simulink model "PIC32MZ_EF_CuriosityBoard_SHT1x_ExtMode"  (R2016b)
settings: Solver=FixedStepDiscrete  StartTime=0.0  StopTime=inf  FixedStep=0.01  RelTol=1e-3
undefined symbols (not defined in the file or in its folder): A14, A15, B0, B1, B5, C2, C3, D1, D2, D3, DiscIntNeverNeededParam, F5, Max, ms, NumBits1, NumBits2, OC3max, OC4max, OC5max, Pin, Resol, Timer, us
libraries: MCHP_Blockset x14, simulink x6
settings Model: SimulationMode=external  ExtModeBatchMode=on  ExtModeTrigDuration=1  Creator=M91449  LastModifiedBy=Lubin Kerhuel
settings OptimizationCC: DefaultParameterBehavior=Inlined  UseSpecifiedMinMax=on  ZeroExternalMemoryAtStartup=off  ZeroInternalMemoryAtStartup=off  NoFixptDivByZeroProtection=on  EfficientFloat2IntCast=on
settings DebuggingCC: ParameterTunabilityLossMsg=error
settings HardwareCC: ProdBitPerPointer=32  ProdBitPerSizeT=32  ProdBitPerPtrDiffT=32  ProdLargestAtomicInteger=Integer  ProdWordSize=32  ProdLongLongMode=on  ProdHWDeviceType=Generic->Custom
settings ModelReferenceCC: ModelReferenceNumInstancesAllowed=Single
settings RTWCC: SystemTargetFile=MCHP_pic32_stf.tlc  TemplateMakefile=MCHP_pic32.tmf  Description=Microchip Embedded Target PIC32 (real-time)  GenerateReport=on  IncludeHyperlinkInReport=on  LaunchReport=on  GenerateTraceInfo=on  GenerateTraceReport=on  GenerateTraceReportSl=on  GenerateTraceReportSf=on  GenerateTraceReportEml=on
settings CodeAppCC: ForceParamTrailComments=on  IgnoreCustomStorageClasses=off  MaxIdLength=255  OperatorAnnotations=on  SimulinkDataObjDesc=on  SFDataObjDesc=on  MATLABFcnDesc=on  InsertBlockDesc=on  MATLABSourceComments=on
settings STFCustomTargetCC: TargetLibSuffix=_lib.a  TargetLangStandard=C99 (ISO)  IncludeMdlTerminateFcn=off  CombineOutputUpdateFcns=on  CombineSignalStateStructs=on  ERTCustomFileBanners=on  SupportContinuousTime=off  RemoveResetFunc=on  MATLABClassNameForMDSCustomization=Simulink.SoftwareTarget.ERTCustomization  GRTInterface=off  SystemTargetFile=MCHP_pic32_stf.tlc
settings ERTTargetCC: TargetLibSuffix=_lib.a  TargetLangStandard=C99 (ISO)  ParMdlRefBuildCompliant=off  CompOptLevelCompliant=off  ConcurrentExecutionCompliant=off  IncludeMdlTerminateFcn=off  CombineSignalStateStructs=on  ERTFirstTimeCompliant=off  SupportNonInlinedSFcns=on  ModelStepFunctionPrototypeControlCompliant=off  CPPClassGenCompliant=off  UseToolchainInfoCompliant=off  ExtMode=on  ExtModeStaticAllocSize=512  ExtModeMexFile=ext_serial_win32_comm_no_acks  ExtModeMexArgs=1 9 115200  InlinedParameterPlacement=NonHierarchical  ERTSrcFileBannerTemplate=MCHP_dsPIC_code_template.cgt  ERTHdrFileBannerTemplate=MCHP_dsPIC_code_template.cgt  ERTDataSrcFileTemplate=MCHP_dsPIC_code_template.cgt  ERTDataHdrFileTemplate=MCHP_dsPIC_code_template.cgt  ERTCustomFileTemplate=MCHP_main.tlc

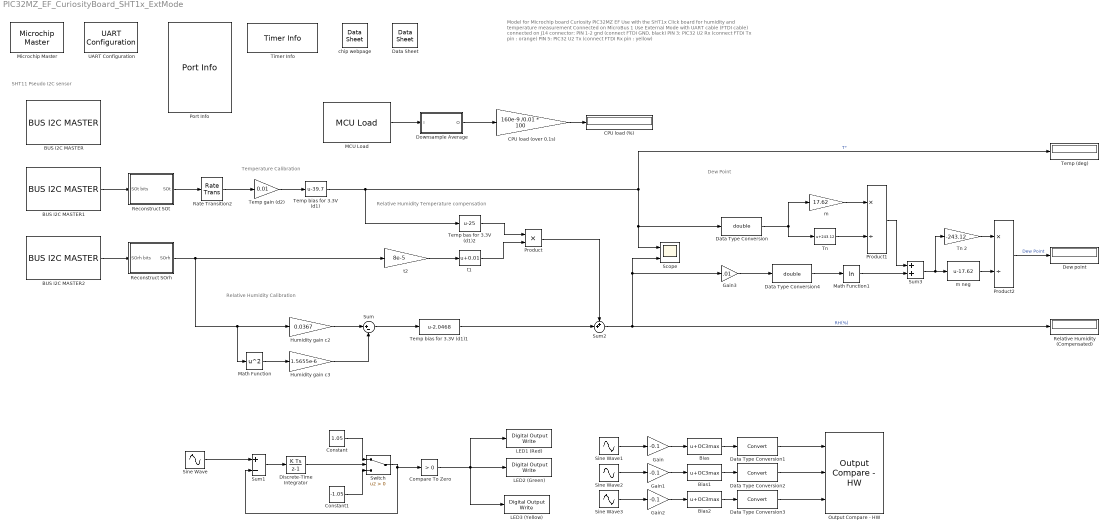
== system PIC32MZ_EF_CuriosityBoard_SHT1x_ExtMode ==
  note: Model for Microchip board Curiosity PIC32MZ EF
      | Use with the SHT1x Click board for humidity and temperature measurement
      | Connected on MicroBus 1
      |
      | Use External Mode with UART cable (FTDI cable) connected on J14 connector:
      | PIN 1-2 gnd (connect FTDI GND, black)
      | PIN 3: PIC32 U2 Rx (connect FTDI Tx pin : orange)
      | PIN 5: PIC32 U2 Tx (connect FTDI Rx pin : yellow)
  note: SHT11 Pseudo I2C sensor
  note: Dew Point
  note: Relative Humidity Temperature compensation
  note: Relative Humidity Calibration
  note: Temperature Calibration
  BUS I2C MASTER : MCHP_Blockset/BUS I2C/BUS I2C MASTER  I2CRef=1  I2C_IntPriority=5  I2Csequence_txt="Initial-Configuration$     ---     $Start    % SHT11 humidity sensor does not use standard I2C protocol$Stop$Start$Write Data (x1)  Write:{[0x03]}      % Start temperature meas (14 bit, might take up to 320ms)$     ---         % Must wait 320ms (sensor pull down SDA line when done)"  I2Csequence_num=[BFF0000000000000 40E0000000000000 40F86A0000000000 40F8650105EF3846]$4070000000000000$[3FF0000000000000 40E0000000000000 40F86A0000000000 40F8650105EF3846]$[4000000000000000 40E0000000000000 40F86A0000000000 40F8650105EF3846]$[3FF0000000000000 40E0000000000000 40F86A0000000000 40F8650105EF3846]$[4050000000000000 3FF0000000000000 0000000000000000 4008000000000000]$4070000000000000  InitialConfigurationNum=0  PIN_SDA_TXT=A15 / Pin[67]  PIN_SCL_TXT=A14 / Pin[66]  S_INPUT="[5  5]"  S_OUTPUT=[5]  S_INPUT_Size="[2  2]"  S_OUTPUT_Size=[4]  BlockingMode=off  SequenceCompleted=off  SampleTime=[1 ]  MCHP_MASTERLINK=PIC32MZ_EF_CuriosityBoard_SHT1x_ExtMode/Microchip Master  MCHP_PORT={I2C 1 Clock}{SCL1}13:0:A14;{I2C 1 SDA}{SDA1}13:0:A15;  ORDERING=0
  BUS I2C MASTER1 : MCHP_Blockset/BUS I2C/BUS I2C MASTER  I2CRef=1  I2C_IntPriority=5  I2Csequence_txt="Initial-Configuration$     ---     $Read Data (x3)  Read:{Out 3}    % Read 14 bit temperature (0.01 deg), last byte is CRC$Stop$Start    % Start measurement for humidity$Stop$Start$Write Data (x1)  Write:{[0x05]}      % Must wait up to 80 ms (12 bit resolution)"  I2Csequence_num=[BFF0000000000000 40E0000000000000 40F86A0000000000 40F8650105EF3846]$4070000000000000$[4060000000000000 4008000000000000]$[4000000000000000 40E0000000000000 40F86A0000000000 40F8650105EF3846]$[3FF0000000000000 40E0000000000000 40F86A0000000000 40F8650105EF3846]$[4000000000000000 40E0000000000000 40F86A0000000000 40F8650105EF3846]$[3FF0000000000000 40E0000000000000 40F86A0000000000 40F8650105EF3846]$[4050000000000000 3FF0000000000000 0000000000000000 4014000000000000]  InitialConfigurationNum=0  PIN_SDA_TXT=A15 / Pin[67]  PIN_SCL_TXT=A14 / Pin[66]  S_INPUT="[5  5]"  S_OUTPUT=[5]  S_INPUT_Size="[2  2]"  S_OUTPUT_Size=[4]  BlockingMode=off  SequenceCompleted=off  SampleTime=[1 0.640]  MCHP_MASTERLINK=PIC32MZ_EF_CuriosityBoard_SHT1x_ExtMode/Microchip Master  MCHP_PORT={I2C 1 Clock}{SCL1}13:0:A14;{I2C 1 SDA}{SDA1}13:0:A15;  ORDERING=0
  BUS I2C MASTER2 : MCHP_Blockset/BUS I2C/BUS I2C MASTER  I2CRef=1  I2C_IntPriority=5  I2Csequence_txt="Initial-Configuration$     ---     $Read Data (x3)  Read:{Out 3}    % Read humidity$Stop"  I2Csequence_num=[BFF0000000000000 40E0000000000000 40F86A0000000000 40F8650105EF3846]$[4070000000000000]$[4060000000000000 4008000000000000]$[4000000000000000 40E0000000000000 40F86A0000000000 40F8650105EF3846]  InitialConfigurationNum=0  PIN_SDA_TXT=A15 / Pin[67]  PIN_SCL_TXT=A14 / Pin[66]  S_INPUT="[5  5]"  S_OUTPUT=[5]  S_INPUT_Size="[2  2]"  S_OUTPUT_Size=[4]  BlockingMode=off  SequenceCompleted=off  SampleTime=[1 .800]  MCHP_MASTERLINK=PIC32MZ_EF_CuriosityBoard_SHT1x_ExtMode/Microchip Master  MCHP_PORT={I2C 1 Clock}{SCL1}13:0:A14;{I2C 1 SDA}{SDA1}13:0:A15;  ORDERING=0
  Bias : Bias  Bias=OC3max
  Bias1 : Bias  Bias=OC3max
  Bias2 : Bias  Bias=OC3max
  CPU load (over 0.1s) : Gain  Gain=160e-9 /0.01 * 100  OutDataTypeStr=double
  CPU load (%) : Display
  Compare To Zero : simulink/Logic and Bit Operations/Compare To Zero  relop=>  OutDataTypeStr=boolean
  Constant : Constant  Value=1.05
  Constant1 : Constant  Value=-1.05
  Data Sheet : MCHP_Blockset/System Info/Data Sheet  DOC_Type=datasheet  DOC_MCHP_Id=32MZ2048EFM100_datasheet  DOC_FilePath=C:\Users\M91449\AppData\Local\Temp\PIC32MZ-EF- Family-DS60001320F.pdf  DOC_FileLastCheckTime="[2019              8             26             15             22         57.115]"  cpy_MCHP_Id=32MZ2048EFM100  MCHP_MASTERLINK=PIC32MZ_EF_CuriosityBoard_SHT1x_ExtMode/Microchip Master
      settings: AttributesFormatString=%<cpy_MCHP_Id>
  Data Type Conversion : DataTypeConversion  OutDataTypeStr=double
  Data Type Conversion1 : DataTypeConversion
  Data Type Conversion2 : DataTypeConversion
  Data Type Conversion3 : DataTypeConversion
  Data Type Conversion4 : DataTypeConversion  OutDataTypeStr=double
  Dew point : Display
  Discrete-Time Integrator : DiscreteIntegrator  gainval=1  InitialConditionSetting=State (most efficient)  SampleTime=-1  ICPrevOutput=DiscIntNeverNeededParam  ICPrevScaledInput=DiscIntNeverNeededParam
  Downsample Average : Subsystem  mask{InputSampleTime=.01, DownSample=100}
      mask prompts: InputSampleTime "Input sample time"; DownSample "DownSample Factor"
      mask Display: disp([ 'DwnSmp\n1/' get_param(gcb,'DownSample')]);
  Gain : Gain  Gain=-0.1
  Gain1 : Gain  Gain=-0.1
  Gain2 : Gain  Gain=-0.1
  Gain3 : Gain  Gain=.01  OutMin=[0]  OutMax=[1]  OutDataTypeStr=fixdt(1,32)
  Humidity gain c2 : Gain  Gain=0.0367  OutMax=2^16*0.0367  OutDataTypeStr=fixdt(1,32)
  Humidity gain c3 : Gain  Gain=1.5655e-6  OutMax=2^32*1.5655e-6  OutDataTypeStr=fixdt(0,32)
  LED1 (Red) : MCHP_Blockset/Digital IO/Digital Output Write  PORT=Dynamic Options  PORT_TXT="E   [ 0 : 9 ]"  PIN=3  PACK=off  SIMULTANEOUS=off  ORDERING=None  SampleTime=-1  MCHP_PORT={Digital Out}{DOU}1:1:E3;  MCHP_MASTERLINK=PIC32MZ_EF_CuriosityBoard_SHT1x_ExtMode/Microchip Master
  LED2 (Green) : MCHP_Blockset/Digital IO/Digital Output Write  PORT=Dynamic Options  PORT_TXT="E   [ 0 : 9 ]"  PIN=4  PACK=off  SIMULTANEOUS=off  ORDERING=None  SampleTime=-1  MCHP_PORT={Digital Out}{DOU}1:1:E4;  MCHP_MASTERLINK=PIC32MZ_EF_CuriosityBoard_SHT1x_ExtMode/Microchip Master
  LED3 (Yellow) : MCHP_Blockset/Digital IO/Digital Output Write  PORT=Dynamic Options  PORT_TXT="E   [ 0 : 9 ]"  PIN=6  PACK=off  SIMULTANEOUS=off  ORDERING=None  SampleTime=-1  MCHP_PORT={Digital Out}{DOU}1:1:E6;  MCHP_MASTERLINK=PIC32MZ_EF_CuriosityBoard_SHT1x_ExtMode/Microchip Master
  MCU Load : MCHP_Blockset/Profiling/MCU Load  MCULoadPin=Dynamic Options  MCULoadPin_TXT=F5 / Pin[65]  MCULoadMeasure=on  TIMER_Resolution=Dynamic Options  TIMER_Resolution_TXT="Resol: 0.16(us)  -  Max: 10.5(ms)"  MCHP_PORT={MCU Load Pin}{MCU_Load}0:1:F5;  MCHP_TIMER_REQUEST={MCU_Load}{MCU_Load}21:5:0:0:[]:1048576;  MCHP_TIMER_RESULT=[4 65535 ]  MCHP_MASTERLINK=PIC32MZ_EF_CuriosityBoard_SHT1x_ExtMode/Microchip Master  MCHP_COMPILED_INFO="CompiledSampleTime= [0.01   0 ];CompiledInportDataTypes=[ ];CompiledInportDataWidth=[];"  Info="Timer 4:  Resol: 160(ns)  -  Max: 10.4858(ms)"  SampleTime=.01
  Math Function : Math  Operator=square  OutDataTypeStr=Inherit: Inherit via internal rule
  Math Function1 : Math  Operator=log  OutDataTypeStr=Inherit: Inherit via internal rule
  Microchip Master : MCHP_Blockset/System Configuration/Microchip Master  Priority=1  PICREF=32MZ2048EFM100  TIMESTEP_REF="Timer  ( 0.01s )"  BUSYFLAG=Dynamic Options  BUSYFLAG_TXT=None  PWRTEN=Not used  BOREN=Disable  BODENV=2.7V  BORV=Not used  FPWRT=128ms  DSBOREN=Enable ZPBOR during Deep Sleep Mode  DSLPBOR=Not used  MCLRE=Enabled  SMCLR=MCLR pin generates a normal system Reset  PMDL1WAY=Allow only one reconfiguration  RSTPRI=Device will obtain reset instruction from Primary flash  TEMP=Not used  SOSCSRC=Not used  SOSCSEL=Not used  IOL1WAY=Allow only one reconfiguration  ALTVREF=Not used  DISUVREG=Not used  DSSWEN=Not used  LPCFG=Not used  RTCBAT=Not used  VBTBOR=Not used  WUTSEL=Not used  POWERSAVE=off  FNOSC=Primary Osc (HS;EC)  FPR=ECIO w/ PLL 16x  FOSFPR=HS3 w/PLL 16x  FOS=Primary Oscillator  FRANGE=High Range  OSCILLATOR_SELECT=External Clock  OSCILLATOR_SELECT_spd=External Clock  QUARTZ=24e6  QUARTZ_spd=24e6  POSCGAIN=2x gain setting  POSCBOOST=Boost the kick start of the oscillator  SOSCGAIN=2x gain setting  SOSCBOOST=Boost the kick start of the oscillator  ACTIV_PLL=on  ACTIV_PLL_spd=on  MIPS_DESIRED=200e6  MIPS_DESIRED_spd=200e6  FPLLMUL=Not used  FPLLIDIV=3x Divider  POSCFREQ=Not used  POSCMD=Primary Oscillator Disabled  POSCMOD=External clock mode  MIPS=199.99999999999997 * 1e6  ACLKCON=Optimized for PWM resolution & ADC conversion speed  ACLKCON_spd=Optimized for PWM resolution & ADC conversion speed  FPLLODIV=2x Divider  PLLKEN=Clock switch to PLL source will wait until the PLL lock signal is valid.  FCKSM=Clock Switch Enabled; FSCM Enabled  FCKSMEN=Sw Disabled; Mon Disabled  IESO=Enabled  DSWDTPS=1:2^36  FWDTEN=Disable  FWDTWINSZ=Window size is 25%  FWPSA=1:512  FWPSA0=1:128  FWPSB=1:16  WDT=Disable  WDTPOST=1:32768  WDTPRE=1:128  WDTPS=1:1048576  WINDIS=Watchdog Timer is in non-Window mode  WWDTEN=Non-Window mode  DSWDTEN=Enable DSWDT during Deep Sleep Mode  DSWDTOSC=Select LPRC as DSWDT Reference clock  FPBDIV=Not used  FSOSCEN=Disable Secondary Oscillator  LPRCSEL=Not used  OSCIOFCN=Not used  OSCIOFNC=Disable  LVRCFG=Not used  PLL_96MHZ=Not used  PLL96MHZ=Not used  PLLDIV=Not used  WDTCLK=Not used  WDTCMX=Not used  WDTWIN=Watchdog Window is 25% of WDT period  XTCFG=24-32 MHz crystals  XTBST=Boost the kick-start  APL=Aux Flash Code protect is disabled  APLK=Aux Flash Write Protection or Code Protection is Enabled  AWRP=Aux Flash may be written  BSS=No Boot program Flash segment  BWP=Not used  BWRP=Boot Segment may be written  CP=Protection Disabled  EBS=No Boot EEPROM  ESS=No Segment Data EEPROM  GCP=General Segment Code protect is Disabled  GSS=User program memory is not code-protected  GSS0=Not used  GSSK=General Segment Write Protection or Code Protection is Enabled  GWRP=General Segment may be written  PWP=Not used  RBS=No Boot RAM  RSS=No Secure RAM  SSS=No Secure Segment  SWRP=Secure segment may be written  WPCFG=Not used  WPDIS=Not used  WPEND=Not used  WPFP=Not used  ICESEL=Communicate on PGEC2/PGED2  ICS=Communicate on PGEC1 and PGED1  JTAGEN=Disable  COE=Not used  RES=Not used  DEBUG=Debugger is disabled  BACKBUG=Not used  BKBUG=Not used  ALTI2C=I2C mapped to SDA1/SCL1 pins  ALTI2C1=I2C1 mapped to SDA1/SCL1 pins  ALTI2C2=I2C2 mapped to SDA2/SCL2 pins  ALTI2C3=I2C3 mapped to SDA3/SCL3 pins  ALTQIO=QEA1; QEB1; INDX1 are selected as inputs to QEI1  ALTSS1=SS1A is selected as the I/O pin for SPI1  CMPPOL0=Hysteresis is applied to falling edge  CMPPOL1=Hysteresis is applied to falling edge  FCANIO=Not used  FETHIO=Default Ethernet I/O  FMIIEN=MII Enabled  FSRSSEL=Not used  FUSBIDIO=Controlled by the USB Module  FVBUSONIO=Not used  HPOL=PWM module high side output pins have active-high output polarity  HYST0=45 mV Hysteresis  HYST1=45 mV Hysteresis  I2C1SEL=Not used  LPOL=PWM module low side output pins have active-high output polarity  PWMPIN=PWM module pins controlled by PORT register at device Reset  RTCOSC=Not used  UPLLEN=USB PLL Disabled  UPLLIDIV=Not used  ATMOD8=Not used  ALTPMP=Not used  I2C2SEL=Not used  ALTADREF=Not used  ALTCVREF=Not used  PWMLOCK=PWM registers may be written without key sequence  INT_PRIORITY_DMA=0  MCHP_TIMER_REQUEST={Time Step}{TS}0:2:3:1:[]:999999.9999999999;  MCHP_TIMER_RESULT=[3 62498.999999999993 ]  MCHP_PLLRegisters="[19988993         0     16386         1        -1]"  MCHPVAR=MCHP.fcy.MIPS=MCHP_Fun.Hex2num('41A7D783FFFFFFFF');MCHP.fcy.SYSCLK=MCHP_Fun.Hex2num('41A7D783FFFFFFFF');MCHP.fcy.ADC=MCHP_Fun.Hex2num('4197D783FFFFFFFF');MCHP.fcy.Comparator=MCHP_Fun.Hex2num('4197D783FFFFFFFF');MCHP.fcy.I2C=MCHP_Fun.Hex2num('4197D783FFFFFFFF');MCHP.fcy.SPI=MCHP_Fun.Hex2num('4197D783FFFFFFFF');MCHP.fcy.UART=MCHP_Fun.Hex2num('4197D783FFFFFFFF');MCHP.fcy.Timers=MCHP_Fun.Hex2num('4197D783FFFFFFFF');MCHP.fcy.OC=MCHP_Fun.Hex2num('4197D783FFFFFFFF');MCHP.fcy.IC=MCHP_Fun.Hex2num('4197D783FFFFFFFF');MCHP.fcy.Ports=MCHP_Fun.Hex2num('41A7D783FFFFFFFF');MCHP.fcy.QEI=MCHP_Fun.Hex2num('4197D783FFFFFFFF');MCHP.PowerSave=0;MCHP.TimeStepFactor=MCHP_Fun.Hex2num('3FF0000000000001');MCHP.TimeStep_Timer=3;MCHP.NTIMERS=9;MCHP.id.name='32MZ2048EFM100';MCHP.id.N=reshape([32 2048 100],1,3);MCHP.id.L=reshape({ 'MZ','EFM',''},1,3);MCHP.id.Arch=4;MCHP.periph.PPS.reg_RPINRx=reshape(MCHP_Fun.Hex2num('[]'),0,0);MCHP.PPS.PIC32.PeriphInput_ppsGroup=reshape({ 'INT3','T2CK','T6CK','IC3','IC7','U1RX','U2CTS','U5RX','U6CTS','SDI1','SDI3','SDI5','SS6_in','REFCLKI1','','','','','','','','','','','','','','','','','','','INT4','T5CK','T7CK','IC4','IC8','U3RX','U4CTS','','','SDI2','SDI4','','C1RX','REFCLKI4','','','','','','','','','','','','','','','','','','','INT2','T3CK','T8CK','IC2','IC5','IC9','U1CTS','U2RX','U5CTS','SS1_in','SS3_in','SS5_in','C2RX','','','','','','','','','','','','','','','','','','','','INT1','T4CK','T9CK','IC1','IC6','','U3CTS','U4RX','U6RX','SS2_in','SDI6','OCFA','','REFCLKI3','','','','','','','','','','','','','','','','','',''},1,128);MCHP.PPS.PIC32.PeriphOutputCode=reshape({ 'NoConnect','U3TX','U4RTS','3','4','SDO1','SDO2','SDO3','8','SDO5','SS6_out','OC3','OC6','REFCLKO4','C2OUT','C1TX','16','17','18','19','20','21','22','23','24','25','26','27','28','29','30','31','NoConnect','U1TX','U2RTS','U5TX','U6RTS','SDO1','SDO2','SDO3','SDO4','SDO5','10','OC4','OC7','13','14','REFCLKO1','16','17','18','19','20','21','22','23','24','25','26','27','28','29','30','31','NoConnect','U3RTS','U4TX','3','U6TX','SS1_out','6','SS3_out','SS4_out','SS5_out','SDO6','OC5','OC8','13','C1OUT','REFCLKO3','16','17','18','19','20','21','22','23','24','25','26','27','28','29','30','31','NoConnect','U1RTS','U2TX','U5RTS','U6TX','5','SS2_out','7','SDO4','11','SDO6','OC2','OC1','OC9','14','C2TX','16','17','18','19','20','21','22','23','24','25','26','27','28','29','30','31'},1,128);MCHP.PPS.PIC32.PinInputCode=reshape({ 'D2','G8','F4','D10','F1','B9','B10','C14','B5','','C1','D14','G1','A14','D6','','D3','G7','F5','D11','F0','B1','E5','C13','B3','','C4','D15','G0','A15','D7','','D9','G6','B8','B15','D4','B0','E3','B7','','F12','D12','F8','C3','E9','','','D1','G9','B14','D0','','B6','D5','B2','F3','F13','','F2','C2','E8','',''},1,64);MCHP.Rx=reshape([17 25 -1 71 91 85 88 -1 -1 -1 -1 38 24 6 76 94 86 87 -1 -1 -1 -1 59 23 7 77 98 57 -1 -1 -1 -1 -1 60 22 8 78 99 56 -1 -1 -1 -1 -1 61 21 9 81 100 64 -1 -1 -1 -1 -1 2 20 -1 82 3 65 -1 -1 -1 -1 -1 89 26 -1 -1 4 -1 10 -1 -1 -1 -1 90 27 -1 -1 5 -1 11 -1 -1 -1 -1 -1 32 -1 -1 18 58 12 -1 -1 -1 -1 28 33 -1 68 19 -1 16 -1 -1 -1 -1 29 34 -1 69 -1 -1 -1 -1 -1 -1 -1 -1 35 -1 70 -1 -1 -1 -1 -1 -1 -1 -1 41 49 79 -1 40 96 -1 -1 -1 -1 -1 42 72 80 -1 39 97 -1 -1 -1 -1 66 43 73 47 -1 -1 95 -1 -1 -1 -1 67 44 50 48 -1 -1 1 -1 -1 -1 -1],11,16);MCHP.ADC.ANtype=reshape([0 0],1,2);MCHP.ADC.ADCONx=reshape([0 0 0 0 0 0],1,6);MCHP.ADC.ADCHS_0=reshape([0 0],1,2);MCHP.ADC.Flags=reshape([-1 0],1,2);MCHP.ADC.Buffer=reshape([-1 -1],1,2);MCHP.ADC.port=reshape([16 17 18 19 20 26 27 28 29 30 31 105 104 103 102 71 70 69 68 36 35 34 33 111 0 72 73 9 10 1 93 92 62 63 5 -1 -1 -1 -1 -1 -1 -1 -1 -1 -1 21 22 23 24 25 -1 -1 -1 -1 -1 -1 -1],1,57);MCHP.ADC.port_ALT=reshape([-1 -1 -1 -1],1,4);MCHP.ADC.port_VrefP=10;MCHP.ADC.port_VrefM=9;MCHP.ADC.port_AVdd=-1;MCHP.ADC.port_AVss=-1;MCHP.ADC.ADCDATA=reshape([1 1 1 1 1 1 1 1 1 1 1 1 1 1 1 1 1 1 1 1 1 1 1 1 1 1 1 1 1 1 1 1 1 1 1 0 0 0 0 0 0 0 0 1 1 0 0 0 0 0 0 0 0 0 0 0 0],1,57);MCHP.ADC.HS_SAR.TRGSRC=reshape([0 0 0 0 0 0 0 0 0 0 0 0 0 0 0 0 0 0 0 0 0 0 0 0 0 0],1,26);MCHP.ADC.HS_SAR.nFilters=0;MCHP.ADC.HS_SAR.nDedicatedCore=0;MCHP.ADC.HS_SAR.CALIBRATION=0;MCHP.ADC.HS_SAR.ADCON1L=-1;MCHP.ADC.HS_SAR.ADC_Class3_idxStart=12;MCHP.memory.RAM=0;MCHP.memory.RAM_XBegin=-1;MCHP.memory.RAM_YBegin=-1;MCHP.memory.RAM_dma=reshape([-1 -1],1,2);MCHP.memory.FLASH_ECC=0;MCHP.DMA.Num=8;MCHP.DMA.CNTmax=65535;MCHP.QEI.QEICONx=reshape([-1 -1 -1 -1 -1 -1],1,6);MCHP.QEI.QEItype=-1;MCHP.QEI.Port_QEI_INDX=reshape([-1 -1],1,2);MCHP.QEI.Port_QEI_QEA=reshape([-1 -1],1,2);MCHP.QEI.Port_QEI_QEB=reshape([-1 -1],1,2);MCHP.QEI.Port_QEI_UPDN=reshape([-1 -1],1,2);MCHP.INT.Port=reshape([48 32767 32767 32767 32767],1,5);MCHP.PWM_HS.Flags=reshape([0 0 0],1,3);MCHP.PWM.port_FLT=reshape([-1 -1 -1 -1 -1 -1 -1 -1 -1 -1 -1 -1 -1 -1 -1 -1 -1 -1 -1 -1 -1 -1 -1 -1 -1 -1 -1 -1 -1 -1 -1 -1 -1],1,33);MCHP.PWM.PWMRef=-1;MCHP.PWM.Flag=0;MCHP.PWM.Port_PWM_l=reshape([-1 -1 -1 -1 -1 -1 -1 -1 -1 -1 -1 -1 -1 -1 -1 -1 -1 -1 -1 -1 -1 -1 -1 -1],2,12);MCHP.PWM.Port_PWM_h=reshape([-1 -1 -1 -1 -1 -1 -1 -1 -1 -1 -1 -1 -1 -1 -1 -1 -1 -1 -1 -1 -1 -1 -1 -1],2,12);MCHP.PWM_HS_FEP.nEVTOUT=-1;MCHP.IC.Port=reshape([32767 32767 32767 32767 32767 32767 32767 32767 32767 0 0 0 0 0 0 0],1,16);MCHP.IC.type=0;MCHP.OC.Port=reshape([32767 32767 32767 32767 32767 32767 32767 32767 32767 0 0 0 0 0 0 0],1,16);MCHP.OC.type=0;MCHP.CN.Port=reshape([-1 -1 -1 -1 -1 -1 -1 -1 -1 -1 -1 -1 -1 -1 -1 -1 -1 -1 -1 -1 -1 -1 -1 -1 -1 -1 -1 -1 -1 -1 -1 -1 -1 -1 -1 -1 -1 -1 -1 -1 -1 -1 -1 -1 -1 -1 -1 -1 -1 -1 -1 -1 -1 -1 -1 -1 -1 -1 -1 -1 -1 -1 -1 -1 -1 -1 -1 -1 -1 -1 -1 -1 -1 -1 -1 -1 -1 -1 -1 -1 -1 -1 -1 -1 -1],1,85);MCHP.CN.PullUp=reshape([50943 65535 61470 65087 1023 12607 62403 0 0 0 0],1,11);MCHP.CN.type=2;MCHP.CN.Flag_PullDown=1;MCHP.SPI.Refs=reshape([1 2 3 4 5 6],1,6);MCHP.SPI.SPIxCON1=MCHP_Fun.Hex2num('41EFF07FFFE00000');MCHP.SPI.SPIxCON2=40843;MCHP.SPI.Port_SDI=reshape([-1 -1 -1 -1 -1 -1],1,6);MCHP.SPI.Port_SDO=reshape([-1 -1 -1 -1 -1 -1],1,6);MCHP.SPI.Port_SCK=reshape([49 102 30 58 93 63],1,6);MCHP.SPI.Port_SS=reshape([-1 -1 -1 -1 -1 -1],1,6);MCHP.I2C.Refs=reshape([1 2 3 4 5],1,5);MCHP.I2C.I2CxCON=8388607;MCHP.I2C.NewRegName=1;MCHP.I2C.Port_SDA=reshape([15 3 82 103 84],1,5);MCHP.I2C.Port_SCL=reshape([14 2 88 104 85],1,5);MCHP.I2C.Port_ASDA=reshape([-1 -1 -1 -1 -1],1,5);MCHP.I2C.Port_ASCL=reshape([-1 -1 -1 -1 -1],1,5);MCHP.I2C.Fuse_Port_SCL_SDA=reshape([-1 -1 -1 -1 -1 -1 -1 -1 -1 -1],2,5);MCHP.I2C.Fuse_Port_ASCL_ASDA=reshape([-1 -1 -1 -1 -1 -1 -1 -1 -1 -1],2,5);MCHP.SCCP.nSCCP=0;MCHP.SCCP.MCCP=reshape([0 0 0 0 0 0 0 0 0],1,9);MCHP.PGA.Port_PGA1P=reshape([-1 -1 -1 -1],1,4);MCHP.PGA.Port_PGA1N=reshape([-1 -1 -1 -1],1,4);MCHP.PGA.Port_PGA2P=reshape([-1 -1 -1 -1],1,4);MCHP.PGA.Port_PGA2N=reshape([-1 -1 -1 -1],1,4);MCHP.PGA.Num=0;MCHP.HS_AnalogComparator.Port_CMP1=reshape([-1 -1 -1 -1],1,4);MCHP.HS_AnalogComparator.Port_CMP2=reshape([-1 -1 -1 -1],1,4);MCHP.HS_AnalogComparator.Port_CMP3=reshape([-1 -1 -1 -1],1,4);MCHP.HS_AnalogComparator.Port_CMP4=reshape([-1 -1 -1 -1],1,4);MCHP.HS_AnalogComparator.PORT_EXTREFx=reshape([-1 -1],1,2);MCHP.HS_AnalogComparator.Port_DACOUTx=reshape([-1 -1],1,2);MCHP.HS_AnalogComparator.Num=0;MCHP.Comp.Port_CVrefin=-1;MCHP.Comp.Port_CVref=-1;MCHP.Comp.Port_CVref1O=-1;MCHP.Comp.Port_CVref2O=-1;MCHP.Comp.Port_CxOUT=reshape([-1 -1 -1 -1 -1],1,5);MCHP.Comp.Port_OAxOUT=reshape([-1 -1 -1 -1 -1],1,5);MCHP.Comp.Port_CxINP=reshape([21 19 -1 -1 -1],1,5);MCHP.Comp.Port_CxINM=reshape([-1 20 103 102 -1 18 105 104 -1 -1 -1 -1 -1 -1 -1 -1 -1 -1 -1 -1],4,5);MCHP.Comp.Port_OAxINP=reshape([-1 -1 -1 -1 -1],1,5);MCHP.Comp.Port_OAxINM=reshape([-1 -1 -1 -1 -1],1,5);MCHP.Comp.nComp=reshape([0 0 0],1,3);MCHP.Comp.OpAmp=0;MCHP.Comp.CVRCON=reshape([32895 0],1,2);MCHP.Comp.CMCON=0;MCHP.CDAC.Port_DACx=reshape([-1 -1 -1],1,3);MCHP.CDAC.nCDAC=0;MCHP.UART.port_Rx=reshape([32767 32767 32767 32767 32767 32767],1,6);MCHP.UART.port_Tx=reshape([32767 32767 32767 32767 32767 32767],1,6);MCHP.UART.port_ARx=reshape([-1 -1],1,2);MCHP.UART.port_ATx=reshape([-1 -1],1,2);MCHP.UART.port_RTS=reshape([32767 32767 32767 32767 32767 32767],1,6);MCHP.UART.port_CTS=reshape([32767 32767 32767 32767 32767 32767],1,6);MCHP.UART.reg_UxMODE=reshape([64511 64511 64511 64511 64511 64511],1,6);MCHP.UART.reg_UxSTA=reshape([33554431 33554431 33554431 33554431 33554431 33554431],1,6);MCHP.modsrc.DOS_02551_cpu_16bit_v7=0;MCHP.modsrc.DOS_01520_wdt_dmt_upb_v1_16bit=0;MCHP.modsrc.DOS_02359a_sent_j2716_upb_v1=0;MCHP.modsrc.DOS_02672_math_progcrc_upb_v1_16bit=0;MCHP.modsrc.DOS_01577_cla_clc_upb_v1=0;MCHP.modsrc.DOS_02915_ecc_v2=0;MCHP.modsrc.DOS_02673_tmr_classa_upb_v1_16bit=0;MCHP.modsrc.DOS_01494_qei_32b_upb_v1_16bit=0;MCHP.modsrc.DOS_02552_msi_upb_v1_Master=0;MCHP.modsrc.DOS_01441_i2c_upb_v1_16bit_TLAH=0;MCHP.modsrc.DOS_03076_uart_protocol_upb_v1_16bit=0;MCHP.modsrc.DOS_01482=0;MCHP.modsrc.DOS_01483_pwm_16bit=0;MCHP.modsrc.DOS_02497_WACV=0;MCHP.modsrc.DOS_02316_nvm_ctrl_v1_16bit=0;MCHP.modsrc.DOS_02653_afe_current_bias_ctrl_upb_v1_16bit=0;MCHP.modsrc.DOS_01459_ptg_pc_upb_v1_16bit=0;MCHP.modsrc.DOS_01512_ccp_mccp_upb_v1_16bit=0;MCHP.modsrc.DOS_02519_dma_sfr_16bit_v2=0;MCHP.modsrc.DOS_02508c11=0;MCHP.modsrc.DOS_02475_dac_pdm_nbit_upb_v1_16bit=0;MCHP.modsrc.DOS_02467_gpio_upb_v1_16bit=0;MCHP.modsrc.DOS_00805_rst_integration_v4=0;MCHP.modsrc.DOS_02659_clk_sib_v12=0;MCHP.modsrc.DOS_02674_wdt_upb_v1_16bit=0;MCHP.modsrc.DOS_01407=0;MCHP.modsrc.DOS_02552_msi_upb_v1_Slave=0;MCHP.modsrc.DOS_02593_amp_pga_ctrl_pb_v2_16bit=0;MCHP.modsrc.DOS_03247_CAN_FD_UPB_V2_16_bit=0;MCHP.modsrc.DOS_01461_afe_ctmu_con_upb_v1_16bit=0;MCHP.modsrc.DOS_02497_WACA=0;MCHP.modsrc.DOS_02478_uart_irda_upb_v1_16bit=0;MCHP.modsrc.DOS_00929=0;MCHP.modsrc.DOS_01198=0;MCHP.modsrc.DOS_03029_WACH=0;MCHP.modsrc.DOS_02949_WACG=0;MCHP.modsrc.DOS_03349_amp_pad_opamp_ctrl_upb_v1=0;MCHP.modsrc.DOS_02237_osc_dco_ctrl_upb_v1_16bit=0;MCHP.modsrc.DOS_02472_ppi_pmp16_upb_v1_16bit=0;MCHP.modsrc.DOS_03994_WAC07=0;MCHP.modsrc.DOS_03662_WACU=0;MCHP.modsrc.DOS_00794=0;MCHP.modsrc.DOS_00931=0;MCHP.modsrc.DOS_00932=0;MCHP.modsrc.DOS_00942=0;MCHP.modsrc.DOS_00938=0;MCHP.modsrc.DOS_00996=0;MCHP.modsrc.DOS_00997=0;MCHP.modsrc.DOS_00998=0;MCHP.modsrc.DOS_00209=0;MCHP.modsrc.DOS_01555_adc=0;MCHP.modsrc.DOS_01293=0;MCHP.modsrc.DOS_00828=0;MCHP.modsrc.DOS_01116=0;MCHP.modsrc.DOS_01017_RPORx=0;MCHP.modsrc.DOS_01017_RPINRx=0;MCHP.modsrc.DOS_01555_nvm_tsmc18_v2_16bit=0;MCHP.modsrc.DOS_00804=0;MCHP.modsrc.DOS_00826=0;MCHP.modsrc.DOS_01555_TLAK_PMDx=0;MCHP.modsrc.DOS_01555_TLAK_INT_=0;MCHP.modsrc.DOS_00933=0;MCHP.modsrc.DOS_01555=0;MCHP.modsrc.DOS_01555_ptg=0;MCHP.modsrc.DOS_00958=0;MCHP.modsrc.DOS_01117_PORTx=0;MCHP.modsrc.DOS_00999=0;MCHP.modsrc.DOS_01041=0;MCHP.modsrc.DOS_00892=0;MCHP.modsrc.DOS_01287_TLAC_PMDx=0;MCHP.modsrc.DOS_01287_TLAC_INT_=0;MCHP.modsrc.DOS_01424=0;MCHP.modsrc.DOS_01332=0;MCHP.modsrc.DOS_01468_PMBA_current_source=0;MCHP.modsrc.DOS_02291_PGA=0;MCHP.modsrc.DOS_01467_Comparator=0;MCHP.modsrc.DOS_01498_TLAY=0;MCHP.modsrc.DOS_00993_PLL_120MHz=0;MCHP.modsrc.DOS_01332_ptg_pc_v1=0;MCHP.modsrc.DOS_00958_pwm_TLAY=0;MCHP.modsrc.TLAY_IOPorts=0;MCHP.modsrc.DOS_00929q=0;MCHP.modsrc.DOS_02415_spi_v5=0;MCHP.modsrc.DOS_RPINRx_16bit_2=0;MCHP.modsrc.DOS_01497_TLAH_PMDx=0;MCHP.modsrc.DOS_02550_TLAL_INT=0;MCHP.modsrc.DOS_00958_pwm_TLAH=0;MCHP.modsrc.DOS_01287_TLAH_INT_=0;MCHP.modsrc.DOS_01113=0;MCHP.modsrc.DOS_01017_PMDx=0;MCHP.modsrc.DOS_00927=0;MCHP.modsrc.DOS_01080=0;MCHP.modsrc.DOS_00794_cpu_16bit_v3=0;MCHP.modsrc.DOS_02192_TLCD_PMDx=0;MCHP.modsrc.DOS_02192_TLCD_INT_=0;MCHP.modsrc.DOS_02192_cmp=0;MCHP.modsrc.DOS_00958_pwm_TLCD=0;MCHP.modsrc.DOS_02192_PORTx_TLCD=0;MCHP.modsrc.DOS_00936=0;MCHP.modsrc.DOS_00995=0;MCHP.modsrc.DOS_00546=0;MCHP.modsrc.DOS_00474=0;MCHP.modsrc.DOS_02481_WACK_MC_Config=0;MCHP.modsrc.DOS_03088_pfm_cache_ocp_v2_WACK=0;MCHP.modsrc.DOS_02819_pfm_ctrl_32bit_upb_v2=1;MCHP.modsrc.DOS_02674_wdt_upb_v1_32bit=1;MCHP.modsrc.DOS_01520_wdt_dmt_upb_v1=1;MCHP.modsrc.DOS_02869_icd_jtag_bvci_upb_v2=0;MCHP.modsrc.DOS_02823_WACJ_clk_cru_upb_v2=0;MCHP.modsrc.DOS_02823_WACN_clk_cru_upb_v2=0;MCHP.modsrc.DOS_01423_RPINRx=1;MCHP.modsrc.DOS_02481_RPORx=0;MCHP.modsrc.DOS_02511_pwr_sib_upb_v1_32bit=0;MCHP.modsrc.DOS_02907_WACN_GP_int_evic_v3=0;MCHP.modsrc.DOS_01500_dma_bvci_v2=1;MCHP.modsrc.DOS_02141_tmr_classa_pb_v2=0;MCHP.modsrc.DOS_02815_tmr_classb_upb_v1=0;MCHP.modsrc.DOS_00740_icap_pb_v1=1;MCHP.modsrc.DOS_00749_ocmp_pb_v1=1;MCHP.modsrc.DOS_01441_i2c_upb_v1_32bit=1;MCHP.modsrc.DOS_01329_spi_pb_v2=1;MCHP.modsrc.DOS_02478_uart_irda_upb_v1_32bit=0;MCHP.modsrc.DOS_03554_cmp_control_upb_v2_32bit=0;MCHP.modsrc.DOS_01445_dac_nbit__control_upb_v1_32bit=0;MCHP.modsrc.DOS_01461_afe_ctmu_con_upb_v1=0;MCHP.modsrc.DOS_01577_cla_clc_upb_v1_32bit=0;MCHP.modsrc.DOS_02467_gpio_ports_upb_v1=1;MCHP.modsrc.DOS_02508_adc_sar_ctrl_upb_v1_PIC32MK=0;MCHP.modsrc.DOS_01261_tmr_rtcc_pb_v2=1;MCHP.modsrc.DOS_01475_lpwr_deep_sleep_ctrl_v2=0;MCHP.modsrc.DOS_EIP_00136_ssx_v1=1;MCHP.modsrc.DOS_02907_WACN_MC_int_evic_v3=0;MCHP.modsrc.DOS_01477_pwm_mc_upb_v1=0;MCHP.modsrc.DOS_01494_qei_32b_upb_v1=0;MCHP.modsrc.DOS_03247_can_fd_upb_v2_pic32mk=0;MCHP.modsrc.DOS_02907_WACK_MC_int_evic_v3=0;MCHP.modsrc.DOS_02514_dfm_strl_sst_upb_v1=0;MCHP.modsrc.DOS_02472_ppi_pmp16_upb_v1=1;MCHP.modsrc.DOS_02813a_usb_otgcore_pb_v3=0;MCHP.modsrc.DOS_02481_WACJ_MC_Config=0;MCHP.modsrc.DOS_02569_pfm_cache_ocp_v1=0;MCHP.modsrc.DOS_02481_WACJ_MC_int_evic_v3=0;MCHP.modsrc.DOS_01459_ptg_pc_upb_v1_SIC=0;MCHP.modsrc.DOS_01427_cmp_control_upb_v1_32bit=0;MCHP.modsrc.DOS_01152_can_bvci_v1=1;MCHP.modsrc.DOS_02787_WACD_Config=1;MCHP.modsrc.DOS_00800_dac_4bit_ctrl_pb_v1=1;MCHP.modsrc.DOS_01539_icd_jtag_pb_v2=1;MCHP.modsrc.DOS_02823_clk_cru_upb_v2=1;MCHP.modsrc.DOS_01423_RPORx=1;MCHP.modsrc.DOS_02907_WACD_int_evic_v3=1;MCHP.modsrc.DOS_00734_uart_irda_pb_v1=1;MCHP.modsrc.DOS_00687_tmr_classa_pb_v1=1;MCHP.modsrc.DOS_00745_tmr_classb_pb_v1=1;MCHP.modsrc.DOS_02508_adc_sar_ctrl_upb_v1=1;MCHP.modsrc.DOS_00866_cmp_control_pb_v2=1;MCHP.modsrc.DOS_01114_eth_bvci_v1=1;MCHP.modsrc.DOS_02831_usb_clk_rst_v2=1;MCHP.modsrc.DOS_01643_pfm_cache_ahb_v2=1;MCHP.modsrc.DOS_EIP_00206r5_sqi_v2=1;MCHP.modsrc.DOS_EIP_00124_usb_hs_otgcore_v1=1;MCHP.modsrc.DOS_EIP_00218_math_rng_ahbs_v2=1;MCHP.modsrc.DOS_EIP_00109_ebi_v1=1;MCHP.modsrc.DOS_EIP_00158_crypto_v1=1;MCHP.PortBase=16;MCHP.PortPrefixe='P';MCHP.clock.PBxDIV=reshape([1 1 1 0 1 -1 0 1],1,8);  MCHP_CRC=15549464  BTMODE=Not used  RES1=Not used  PLLSS=Not used  RES2=Not used  ALTCMPI=Not used  BOREN1=Not used  ALTRB6=Not used  RETCFG=Not used  DFMCY=Not used  BSS2=No Boot Segment  BSEN=No Boot Segment  CWRP=Configuration Segment may be written  CSS=No Protection (other than CWRP)  AIVTDIS=Disable Alternate Vector Table  BSLIM=Not used  WDTEN=Disable  BTSWP=BOOTSWP instruction is disabled  DBCC=No Cross Connection between DAC outputs  CTXT1=Not Assigned  CTXT2=Not Assigned  SEQNUM=Not used  nSEQNUM=Not used  BOREN0=Enabled  DMTIVT=Not used  DMTCNT=2^8 (256)  DMTEN=Dead Man Timer is Disabled and can be enabled by software  ON=Not used  USERID=Not used  RESERVED1=Not used  PGL1WAY=Allow only one reconfiguration  FPLLRNG=5-10 MHz Input  FPLLICLK=POSC is input to the System PLL  FPLLMULT=PLL Multiply by 50  UPLLFSEL=USB PLL input is 24 MHz  DMTINTV=Window/Interval value is 127/128 counter value  WDTSPGM=WDT stops during Flash programming  FDMTEN=Deadman Timer is disabled  TRCEN=Trace features in the CPU are enabled  BOOTISA=Boot code and Exception code is MIPS32  FECCCON=ECC and Dynamic ECC are disabled (ECCCON bits are writable)  EXTDDRSIZE=Not used  FSLEEP=Flash is powered down when the device is in Sleep mode  DBGPER=Allow CPU access to all permission regions  EJTAGBEN=Normal EJTAG functionality  TSEQ=Not used  CSEQ=Not used  RWDTPS=1:1048576  RCLKSEL=Always use LPRC  SWDTPS=1:1048576  DMTIVTL=Not used  DMTIVTH=Not used  DMTCNTL=Not used  DMTCNTH=Not used  DMTDIS=Dead Man Timer is Disabled and can be enabled by software  SMBEN=SMBus input threshold is enabled  SPI2PIN=SPI2 uses I/O remap (PPS) pins  CTXT3=Not Assigned  CTXT4=Not Assigned  MBXM0=Mailbox register configured for Master data read (Slave to Master data transfer)  MBXM1=Mailbox register configured for Master data read (Slave to Master data transfer)  MBXM2=Mailbox register configured for Master data read (Slave to Master data transfer)  MBXM3=Mailbox register configured for Master data read (Slave to Master data transfer)  MBXM4=Mailbox register configured for Master data read (Slave to Master data transfer)  MBXM5=Mailbox register configured for Master data read (Slave to Master data transfer)  MBXM6=Mailbox register configured for Master data read (Slave to Master data transfer)  MBXM7=Mailbox register configured for Master data read (Slave to Master data transfer)  MBXM8=Mailbox register configured for Master data read (Slave to Master data transfer)  MBXM9=Mailbox register configured for Master data read (Slave to Master data transfer)  MBXM10=Mailbox register configured for Master data read (Slave to Master data transfer)  MBXM11=Mailbox register configured for Master data read (Slave to Master data transfer)  MBXM12=Mailbox register configured for Master data read (Slave to Master data transfer)  MBXM13=Mailbox register configured for Master data read (Slave to Master data transfer)  MBXM14=Mailbox register configured for Master data read (Slave to Master data transfer)  MBXM15=Mailbox register configured for Master data read (Slave to Master data transfer)  MBXHSA=MSIxMBXD15 assigned to mailbox handshake protocol block A  MBXHSB=MSIxMBXD15 assigned to mailbox handshake protocol block B  MBXHSC=MSIxMBXD15 assigned to mailbox handshake protocol block C  MBXHSD=MSIxMBXD15 assigned to mailbox handshake protocol block D  MBXHSE=MSIxMBXD15 assigned to mailbox handshake protocol block E  MBXHSF=MSIxMBXD15 assigned to mailbox handshake protocol block F  MBXHSG=MSIxMBXD15 assigned to mailbox handshake protocol block G  MBXHSH=MSIxMBXD15 assigned to mailbox handshake protocol block H  HSAEN=Mailbox data flow control handshake protocol block disabled.  HSBEN=Mailbox data flow control handshake protocol block disabled.  HSCEN=Mailbox data flow control handshake protocol block disabled.  HSDEN=Mailbox data flow control handshake protocol block disabled.  HSEEN=Mailbox data flow control handshake protocol block disabled.  HSFEN=Mailbox data flow control handshake protocol block disabled.  HSGEN=Mailbox data flow control handshake protocol block disabled.  HSHEN=Mailbox data flow control handshake protocol block disabled.  CPRA0=Master core owns pin.  CPRA1=Master core owns pin.  CPRA2=Master core owns pin.  CPRA3=Master core owns pin.  CPRA4=Master core owns pin.  CPRB0=Master core owns pin.  CPRB1=Master core owns pin.  CPRB2=Master core owns pin.  CPRB3=Master core owns pin.  CPRB4=Master core owns pin.  CPRB5=Master core owns pin.  CPRB6=Master core owns pin.  CPRB7=Master core owns pin.  CPRB8=Master core owns pin.  CPRB9=Master core owns pin.  CPRB10=Master core owns pin.  CPRB11=Master core owns pin.  CPRB12=Master core owns pin.  CPRB13=Master core owns pin.  CPRB14=Master core owns pin.  CPRB15=Master core owns pin.  CPRC0=Master core owns pin.  CPRC1=Master core owns pin.  CPRC2=Master core owns pin.  CPRC3=Master core owns pin.  CPRC4=Master core owns pin.  CPRC5=Master core owns pin.  CPRC6=Master core owns pin.  CPRC7=Master core owns pin.  CPRC8=Master core owns pin.  CPRC9=Master core owns pin.  CPRC10=Master core owns pin.  CPRC11=Master core owns pin.  CPRC12=Master core owns pin.  CPRC13=Master core owns pin.  CPRC14=Master core owns pin.  CPRC15=Master core owns pin.  CPRD0=Master core owns pin.  CPRD1=Master core owns pin.  CPRD2=Master core owns pin.  CPRD3=Master core owns pin.  CPRD4=Master core owns pin.  CPRD5=Master core owns pin.  CPRD6=Master core owns pin.  CPRD7=Master core owns pin.  CPRD8=Master core owns pin.  CPRD9=Master core owns pin.  CPRD10=Master core owns pin.  CPRD11=Master core owns pin.  CPRD12=Master core owns pin.  CPRD13=Master core owns pin.  CPRD14=Master core owns pin.  CPRD15=Master core owns pin.  CPRE0=Master core owns pin.  CPRE1=Master core owns pin.  CPRE2=Master core owns pin.  CPRE3=Master core owns pin.  CPRE4=Master core owns pin.  CPRE5=Master core owns pin.  CPRE6=Master core owns pin.  CPRE7=Master core owns pin.  CPRE8=Master core owns pin.  CPRE9=Master core owns pin.  CPRE10=Master core owns pin.  CPRE11=Master core owns pin.  CPRE12=Master core owns pin.  CPRE13=Master core owns pin.  CPRE14=Master core owns pin.  CPRE15=Master core owns pin.  S1FNOSC=Internal Fast RC (FRC) Oscillator with postscaler  S1IESO=Start up with FRC; then switch  S1OSCIOFNC=OSC2 is clock output  S1FCKSM=Both Clock switching and Fail-safe Clock Monitor are disabled  S1PLLKEN=S1PLLKEN_ON  S1RWDTPS=1:1048576  S1RCLKSEL=Always use LPRC  S1WINDIS=Watchdog Timer operates in Non-Window mode  S1WDTWIN=WDT Window is 25% of WDT period  S1SWDTPS=1:1048576  S1FWDTEN=Disable  S1ICS=Communicate on PGC1 and PGD1  S1DEBUG=Not used  S1ISOLAT=The slave can operate (in debug mode) even if the SLVEN bit in the MSI is zero.  S1NOBTSWP=BOOTSWP instruction is disabled  S1ALTI2C1=I2C1 mapped to SDA1/SCL1 pins  S1SPI1PIN=Slave SPI1 uses I/O remap (PPS) pins  S1SSRE=Slave generated resets will reset the Slave Enable Bit in the MSI module  S1MSRE=The master software oriented RESET events (RESET Op-Code; Watchdog timeout; TRAP reset; illegalInstruction) will also cause the slave subsystem to reset.  S1CTXT1=Not Assigned  S1CTXT2=Not Assigned  S1CTXT3=Not Assigned  S1CTXT4=Not Assigned  BORLVL=Not used  BSSO=Not used  MCA=Not used  MAXTEMP=Not used  CFGAN14=Not used  CFGAN15=Not used  S1IOL1WAY=Not used  S1BSSO=Not used  S1BACKBUG=Not used  BISTDIS=mBIST on reset feature disabled  NOBTSWP=BOOTSWP instruction is disabled  S1BISTDIS=Slave BIST on reset feature disabled  S1DMTIVTL=Not used  S1DMTIVTH=Not used  S1DMTCNTL=Not used  S1DMTCNTH=Not used  S1DMTDIS=Slave Dead Man Timer is Disabled and can be enabled by software  BSEQ=Not used  IBSEQ=Not used  SMB3EN=SMBus 3.0 input levels  FUSBIDIO2=USBID pin is controlled by the USB2 module  FVBUSIO2=VBUSON pin is controlled by the USB2 module  FUSBIDIO1=USBID pin is controlled by the USB1 module  FVBUSIO1=VBUSON pin is controlled by the USB1 module  VBATBOREN=Enable ZPBOR during VBAT Mode  FDSEN=Enable DSEN bit in DSCON  BORSEL=BOR trip voltage 2.1v (Non-OPAMP deviced operation)  POSCFGAIN=Gain is G3  POSCAGCDLY=Settling time = 25ms x AGCRNG  POSCAGCRNG=Range 1x  POSCAGC=Automatic Gain Control for Oscillator  FDBGWP=Not used
  Output Compare - HW : MCHP_Blockset/Pulse Input//Output/Output Compare - HW  Channel="[3     4     5]"  Channel_OLD="[3     4     5]"  PIN_OC1_TXT=D1 / Pin[76]  PIN_OC2_TXT=D1 / Pin[76]  PIN_OC3_TXT=B5 / Pin[20]  PIN_OC4_TXT=B1 / Pin[24]  PIN_OC5_TXT=B0 / Pin[25]  PIN_OC6_TXT=Dynamic Options  PIN_OC7_TXT=Dynamic Options  PIN_OC8_TXT=Dynamic Options  PIN_OC9_TXT=Dynamic Options  PIN_OC10_TXT=Dynamic Options  PIN_OC11_TXT=Dynamic Options  PIN_OC12_TXT=Dynamic Options  PIN_OC13_TXT=Dynamic Options  PIN_OC14_TXT=Dynamic Options  PIN_OC15_TXT=Dynamic Options  PIN_OC16_TXT=Dynamic Options  PIN_OCFA_TXT=Dynamic Options  PIN_OCFB_TXT=Dynamic Options  PIN_OCFC_TXT=Dynamic Options  Channel_UP_Down_Periode="[5     5     5]"  PulseTrig=Continuous pulses  InputPeriod=are set to the Max time (constant below)  MaxChannel="[0.001   0.001   0.001]"  MaxChannelUnique=.001  MaxChannelValue="2.^[ 15.610  15.610  15.610]  =>  [49999  49999  49999]"  OCxmax="[49999  49999  49999]"  Timer="[2  2  2]"  evalin_ws=OC3max=MCHP_Fun.Hex2num('40E869E000000000');OC4max=MCHP_Fun.Hex2num('40E869E000000000');OC5max=MCHP_Fun.Hex2num('40E869E000000000');  SampleTime=-1  MCHP_PORT={Output Compare 3}{OC3}7:1:P21;{Output Compare 4}{OC4}7:1:P17;{Output Compare 5}{OC5}7:1:P16;  MCHP_TIMER_REQUEST="{Output Compare 1}{OC1}7:2:3:0:[2  3]:99999.99999999999;{Output Compare 2}{OC2}7:2:3:0:[2  3]:99999.99999999999;{Output Compare 3}{OC3}7:2:3:0:[2  3]:99999.99999999999;"  MCHP_TIMER_RESULT=[2 49999.000000000015 ;2 49999.000000000015 ;2 49999.000000000015 ]  MCHP_MASTERLINK=PIC32MZ_EF_CuriosityBoard_SHT1x_ExtMode/Microchip Master  PIN_OC1=Dynamic Options  PIN_OC2=Dynamic Options  PIN_OC3=Dynamic Options  PIN_OC4=Dynamic Options  PIN_OC5=Dynamic Options  PIN_OC6=Dynamic Options  PIN_OC7=Dynamic Options  PIN_OC8=Dynamic Options  PIN_OC9=Dynamic Options  PIN_OC10=Dynamic Options  PIN_OC11=Dynamic Options  PIN_OC12=Dynamic Options  PIN_OC13=Dynamic Options  PIN_OC14=Dynamic Options  PIN_OC15=Dynamic Options  PIN_OC16=Dynamic Options  PIN_OCFA=Dynamic Options  PIN_OCFB=Dynamic Options  PIN_OCFC=Dynamic Options
  Port Info : MCHP_Blockset/System Info/Port Info  MCHP_MASTERLINK=PIC32MZ_EF_CuriosityBoard_SHT1x_ExtMode/Microchip Master
  Product : Product
  Product1 : Product  Inputs=*/
  Product2 : Product  Inputs=*/
  Rate Transition2 : RateTransition  Integrity=off
  Reconstruct SOrh : Subsystem
  Reconstruct SOt : Subsystem
  Relative Humidity (Compensated) : Display
  Scope : Scope  NumInputPorts=2
  Sine Wave : Sin  Frequency=2*pi*1/5  SampleTime=.01
  Sine Wave1 : Sin  Amplitude=OC3max/2  Bias=OC3max/2  Frequency=2*pi*1/5  SampleTime=.01
  Sine Wave2 : Sin  Amplitude=OC4max/2  Bias=OC4max/2  Frequency=2*pi*1/5  Phase=2*pi/3  SampleTime=.01
  Sine Wave3 : Sin  Amplitude=OC5max/2  Bias=OC5max/2  Frequency=2*pi*1/5  Phase=4*pi/3  SampleTime=.01
  Sum : Sum  Inputs=|+-
  Sum1 : Sum  Inputs=+-
  Sum2 : Sum  Inputs=++|
  Sum3 : Sum
  Switch : Switch  Criteria=u2 > Threshold
  Temp (deg) : Display
  Temp bas for 3.3V (d1)2 : Bias  Bias=-25
  Temp bias for 3.3V (d1) : Bias  Bias=-39.7
  Temp bias for 3.3V (d1)1 : Bias  Bias=-2.0468
  Temp gain (d2) : Gain  Gain=0.01  OutMin=0  OutMax=655.35  OutDataTypeStr=fixdt(1,16)
  Timer Info : MCHP_Blockset/System Info/Timer Info  MCHP_MASTERLINK=PIC32MZ_EF_CuriosityBoard_SHT1x_ExtMode/Microchip Master
  Tn : Bias  Bias=243.12
  Tn 2 : Gain  Gain=-243.12
  UART Configuration : MCHP_Blockset/BUS UART/UART Configuration  UART_REF=2  BAUD_Choice=Dynamic Options  BAUD_Choice_TXT="115200         [+0.01%]"  BAUD_Choice_IR=Dynamic Options  BAUD_Choice_IR_TXT=[]  BAUD_Custom=115200  INT_PRIORITY=0  ALT_IO=on  PIN_RX=Dynamic Options  PIN_RX_TXT=C3 / Pin[8]  PIN_TX=Dynamic Options  PIN_TX_TXT=C2 / Pin[7]  MCHP_PORT="{UART2  Rx}{U2RX}3:0:P35;{UART2  Tx}{U2TX}3:1:P34;"  MCHP_MASTERLINK=PIC32MZ_EF_CuriosityBoard_SHT1x_ExtMode/Microchip Master  MCHP_COM_ExtPil=on  TX_IMPLEMENTATION=Circular Buffer  TX_IMPLEMENTATION_default=Circular Buffer  TX_INT_PRIORITY=3  TX_INT_WHEN=is empty  TX_INT_WHEN_default=is empty & last char is sent  TX_CIRCULAR_SIZE=64  TX_DMA_CHANNEL="0   (Lowest Priority)"  TX_DMA_SIZE=[]  TX_TASK_PROTECTION=Delay tasks (default)  TX_INTERRUPT_PROTECTION=Do not send on conflict (default)  TX_INTERRUPT_PROTECTION_default=Do not send on conflict (default)  RX_IMPLEMENTATION=Circular Buffer  RX_IMPLEMENTATION_default=Circular Buffer  RX_INT_PRIORITY=6  RX_INT_WHEN=is 3/4 fulll (contains 3 data characters)  RX_CIRCULAR_SIZE=64  RX_DMA_CHANNEL=0  RX_DMA_SIZE=0  DuplexMode=Full duplex (default)  PIN_RX_Inv=off  PIN_TX_Inv=off  PIN_RXTX_Inv=off  ParityBit=No parity (default)  StopBit=1 stop bit (default)  IRDA=off  FlowControl=None  PIN_CTS=Dynamic Options  PIN_CTS_TXT=D2 / Pin[77]  PIN_RTS=Dynamic Options  PIN_RTS_TXT=D3 / Pin[78]  InitSequence_chkbox=off  BAUD_Choice_InitSeq=Dynamic Options  BAUD_Choice_InitSeq_TXT="110         [+0.00%]"  BAUD_Choice_IR_InitSeq=Dynamic Options  BAUD_Choice_IR_InitSeq_TXT=0  BAUD_Custom_InitSeq=0  InitSequence='Hello World'
  chip webpage : MCHP_Blockset/System Info/Data Sheet  DOC_Type=www  DOC_MCHP_Id=33FJ64MC802  DOC_FileLastCheckTime=[0 0 0 0 0 0]  cpy_MCHP_Id=32MZ2048EFM100  MCHP_MASTERLINK=PIC32MZ_EF_CuriosityBoard_SHT1x_ExtMode/Microchip Master
      settings: AttributesFormatString=%<cpy_MCHP_Id>
  m : Gain  Gain=17.62
  m neg : Bias  Bias=-17.62
  t1 : Bias  Bias=0.01
  t2 : Gain  Gain=8e-5  OutMax=2^16*8e-5  OutDataTypeStr=fixdt(0,16)
  wires:
  Sine Wave/1 -> Sum1/1
  Discrete-Time Integrator/1 -> Switch/2
  Constant/1 -> Switch/1
  Constant1/1 -> Switch/3
  Switch/1 -> Compare To Zero/1, Sum1/2
  Sum1/1 -> Discrete-Time Integrator/1
  Data Type Conversion1/1 -> Output Compare - HW/1
  Sine Wave1/1 -> Gain/1
  Sine Wave2/1 -> Gain1/1
  Data Type Conversion2/1 -> Output Compare - HW/2
  Sine Wave3/1 -> Gain2/1
  Data Type Conversion3/1 -> Output Compare - HW/3
  Gain/1 -> Bias/1
  Gain1/1 -> Bias1/1
  Gain2/1 -> Bias2/1
  Bias/1 -> Data Type Conversion1/1
  Bias1/1 -> Data Type Conversion2/1
  Bias2/1 -> Data Type Conversion3/1
  Compare To Zero/1 -> LED2 (Green)/1, LED3 (Yellow)/1, LED1 (Red)/1
  BUS I2C MASTER2/1 -> Reconstruct SOrh/1(SOrh bits)
  Reconstruct SOrh/1(SOrh) -> Math Function/1, Humidity gain c2/1, t2/1
  Temp gain (d2)/1 -> Temp bias for 3.3V (d1)/1
  Temp bias for 3.3V (d1)/1 -> Temp (deg)/1, Scope/1, Data Type Conversion/1, Temp bas for 3.3V (d1)2/1  "T°"
  Math Function/1 -> Humidity gain c3/1
  Temp bias for 3.3V (d1)1/1 -> Sum2/2
  Sum/1 -> Temp bias for 3.3V (d1)1/1
  Temp bas for 3.3V (d1)2/1 -> Product/1
  t2/1 -> t1/1
  t1/1 -> Product/2
  Product/1 -> Sum2/1
  Sum2/1 -> Gain3/1, Scope/2, Relative Humidity (Compensated)/1  "RH(%)"
  Reconstruct SOt/1(SOt) -> Rate Transition2/1
  BUS I2C MASTER1/1 -> Reconstruct SOt/1(SOt bits)
  Rate Transition2/1 -> Temp gain (d2)/1
  Humidity gain c2/1 -> Sum/1
  Humidity gain c3/1 -> Sum/2
  MCU Load/1 -> Downsample Average/1(I)
  CPU load (over 0.1s)/1 -> CPU load (%)/1
  Gain3/1 -> Data Type Conversion4/1
  Data Type Conversion4/1 -> Math Function1/1
  Data Type Conversion/1 -> Tn/1, m/1
  m/1 -> Product1/1
  Tn/1 -> Product1/2
  Product1/1 -> Sum3/1
  Math Function1/1 -> Sum3/2
  Sum3/1 -> Tn 2/1, m neg/1
  m neg/1 -> Product2/2
  Tn 2/1 -> Product2/1
  Product2/1 -> Dew point/1  "Dew Point"
  Downsample Average/1(O) -> CPU load (over 0.1s)/1

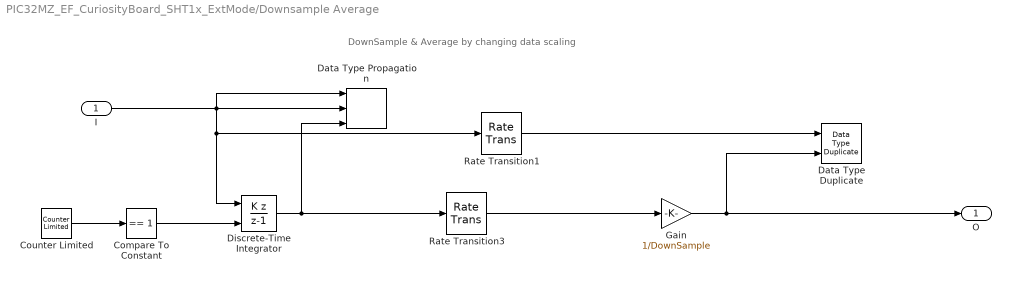
== system PIC32MZ_EF_CuriosityBoard_SHT1x_ExtMode/Downsample Average ==
  note: DownSample & Average by changing data scaling
  I : Inport
  Compare To Constant : simulink/Logic and Bit Operations/Compare To Constant  relop===  const=1  OutDataTypeStr=boolean
  Counter Limited : simulink/Sources/Counter Limited  uplimit=DownSample-1  tsamp=-1
  Data Type Duplicate : DataTypeDuplicate
  Data Type Propagation : simulink/Signal Attributes/Data Type Propagation  PropDataType=fixdt(1, 16)  IfRefDouble=double  IfRefSingle=single  IsSigned=IsSigned1 or IsSigned2  NumBitsBase=NumBits1+NumBits2  NumBitsMult=1  NumBitsAdd=0  NumBitsAllowFinal=1:128  PropScaling=2^-10  ValuesUsedBestPrec=[5 -7]  SlopeBase=Slope1  SlopeMult=1  SlopeAdd=0  BiasBase=Bias1  BiasMult=1  BiasAdd=0
  Discrete-Time Integrator : DiscreteIntegrator  IntegratorMethod=Accumulation: Backward Euler  gainval=1  ExternalReset=sampled level  InitialConditionSetting=State (most efficient)  SampleTime=-1  OutDataTypeStr=Inherit: Inherit via back propagation  ICPrevOutput=DiscIntNeverNeededParam  ICPrevScaledInput=DiscIntNeverNeededParam
  Gain : Gain  Gain=1/DownSample  OutDataTypeStr=Inherit: Inherit via back propagation
  Rate Transition1 : RateTransition  Deterministic=off  OutPortSampleTime=[InputSampleTime * DownSample]
  Rate Transition3 : RateTransition  OutPortSampleTime=[InputSampleTime * DownSample]
  O : Outport
  wires:
  Rate Transition3/1 -> Gain/1
  I/1 -> Discrete-Time Integrator/1, Rate Transition1/1, Data Type Propagation/2, Data Type Propagation/1
  Compare To Constant/1 -> Discrete-Time Integrator/2
  Discrete-Time Integrator/1 -> Data Type Propagation/3, Rate Transition3/1
  Counter Limited/1 -> Compare To Constant/1
  Gain/1 -> Data Type Duplicate/2, O/1
  Rate Transition1/1 -> Data Type Duplicate/1

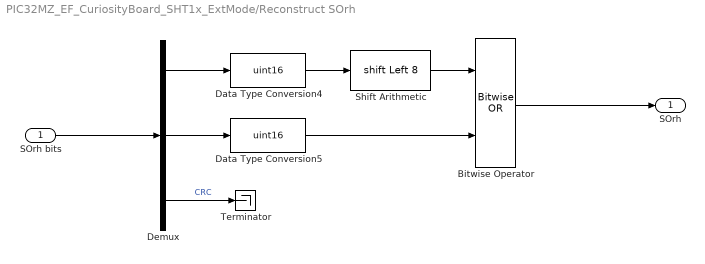
== system PIC32MZ_EF_CuriosityBoard_SHT1x_ExtMode/Reconstruct SOrh ==
  SOrh bits : Inport
  Bitwise Operator : simulink/Logic and Bit Operations/Bitwise Operator  logicop=OR  UseBitMask=off  NumInputPorts=2  BitMask=bin2dec('11011001')  BitMaskRealWorld=Stored Integer
  Data Type Conversion4 : DataTypeConversion  OutDataTypeStr=uint16  ConvertRealWorld=Stored Integer (SI)
  Data Type Conversion5 : DataTypeConversion  OutDataTypeStr=uint16  ConvertRealWorld=Stored Integer (SI)
  Demux : Demux  Outputs=3
  Shift Arithmetic : ArithShift  BitShiftNumber=8  BitShiftDirection=Left
  Terminator : Terminator
  SOrh : Outport
  wires:
  Demux/3 -> Terminator/1  "CRC"
  SOrh bits/1 -> Demux/1
  Shift Arithmetic/1 -> Bitwise Operator/1
  Bitwise Operator/1 -> SOrh/1
  Data Type Conversion5/1 -> Bitwise Operator/2
  Demux/2 -> Data Type Conversion5/1
  Data Type Conversion4/1 -> Shift Arithmetic/1
  Demux/1 -> Data Type Conversion4/1

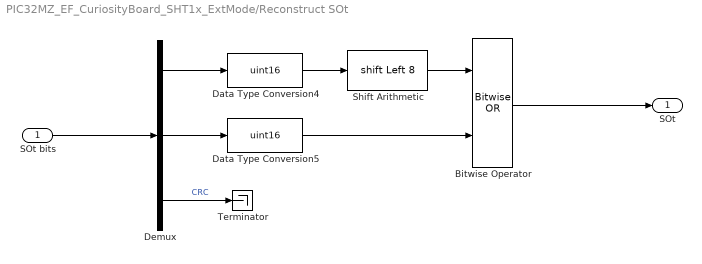
== system PIC32MZ_EF_CuriosityBoard_SHT1x_ExtMode/Reconstruct SOt ==
  SOt bits : Inport
  Bitwise Operator : simulink/Logic and Bit Operations/Bitwise Operator  logicop=OR  UseBitMask=off  NumInputPorts=2  BitMask=bin2dec('11011001')  BitMaskRealWorld=Stored Integer
  Data Type Conversion4 : DataTypeConversion  OutDataTypeStr=uint16  ConvertRealWorld=Stored Integer (SI)
  Data Type Conversion5 : DataTypeConversion  OutDataTypeStr=uint16  ConvertRealWorld=Stored Integer (SI)
  Demux : Demux  Outputs=3
  Shift Arithmetic : ArithShift  BitShiftNumber=8  BitShiftDirection=Left
  Terminator : Terminator
  SOt : Outport
  wires:
  Demux/1 -> Data Type Conversion4/1
  Data Type Conversion4/1 -> Shift Arithmetic/1
  Demux/2 -> Data Type Conversion5/1
  Data Type Conversion5/1 -> Bitwise Operator/2
  Bitwise Operator/1 -> SOt/1
  Shift Arithmetic/1 -> Bitwise Operator/1
  SOt bits/1 -> Demux/1
  Demux/3 -> Terminator/1  "CRC"
